simulink model "W06_3_heading"  (R2024b)
settings: Solver=FixedStepDiscrete  StartTime=0.0  StopTime=inf  FixedStep=0.05  RelTol=1e-3
libraries: ros2lib x5, slpidlib x1
settings Model: Creator=admin  LastModifiedBy=admin

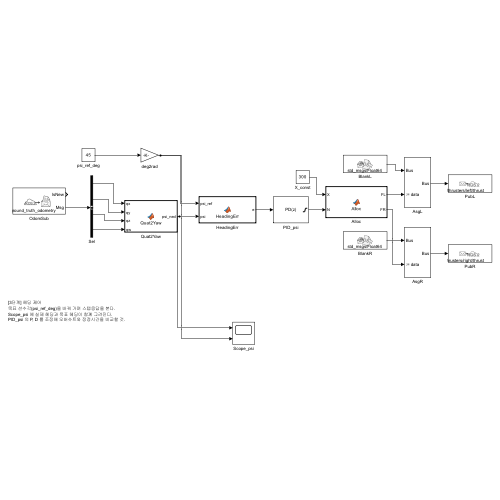
[thumbnail: Simulink's stored preview of the top-level diagram]
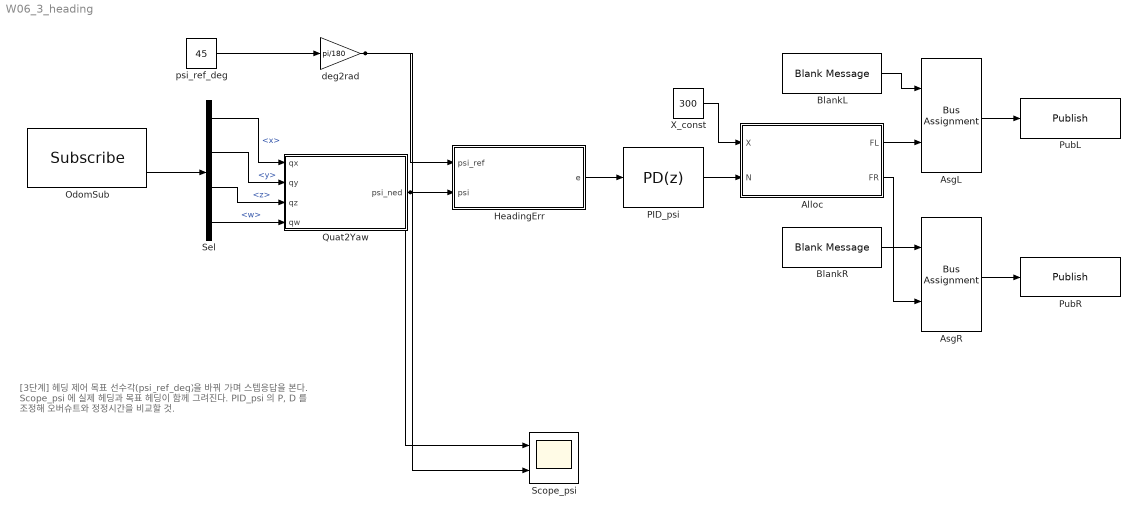
== system W06_3_heading ==
  note: [3단계] 헤딩 제어
      | 목표 선수각(psi_ref_deg)을 바꿔 가며 스텝응답을 본다.
      | Scope_psi 에 실제 헤딩과 목표 헤딩이 함께 그려진다.
      | PID_psi 의 P, D 를 조정해 오버슈트와 정정시간을 비교할 것.
  Alloc : MATLAB Function  TreatAsAtomicUnit=on
  AsgL : BusAssignment  AssignedSignals=data
  AsgR : BusAssignment  AssignedSignals=data
  BlankL : ros2lib/Blank Message  messageClass=Message  entityType=std_msgs/Float64  messageType=std_msgs/Float64  SampleTime=0.05
  BlankR : ros2lib/Blank Message  messageClass=Message  entityType=std_msgs/Float64  messageType=std_msgs/Float64  SampleTime=0.05
  HeadingErr : MATLAB Function  TreatAsAtomicUnit=on
  OdomSub : ros2lib/Subscribe  topicSource=Specify your own  topic=/wamv/sensors/position/ground_truth_odometry  messageType=nav_msgs/Odometry  sampleTime=0.05  QOSHistory=Keep last  QOSDepth=1  QOSReliability=Reliable  QOSDurability=Volatile  QOSDeadline=Inf  QOSLifespan=Inf  QOSLiveliness=Automatic  QOSLeaseDuration=Inf  QOSAvoidROSNamespaceConventions=off
  PID_psi : slpidlib/PID Controller  Controller=PD  Form=Parallel  TimeDomain=Discrete-time  UseExternalTs=off  SampleTime=0.05  IntegratorMethod=Forward Euler  FilterMethod=Forward Euler  ControllerParametersSource=internal  P=800  I=1  UseKiTs=off  D=400  UseExternalDerivativeSource=off  N=100  UseFilter=on  TunerSelectOption=Transfer Function Based (PID Tuner App)  InitialConditionSource=internal  InitialConditionForIntegrator=0  InitialConditionForFilter=0  DifferentiatorICPrevScaledInput=0  ExternalReset=none  TrackingMode=off  Kt=1  LimitOutput=on  SatLimitsSource=internal  UpperSaturationLimit=500  LowerSaturationLimit=-500  LinearizeAsGain=off  AntiWindupMode=none  Kb=1  LimitIntegrator=off  UpperIntegratorSaturationLimit=inf  LowerIntegratorSaturationLimit=-inf  POutMin=[]  POutMax=[]  IOutMin=[]  IOutMax=[]  DOutMin=[]  DOutMax=[]  NOutMin=[]  NOutMax=[]  SumOutMin=[]  SumOutMax=[]  SaturationOutMin=[]  SaturationOutMax=[]  PParamMin=[]  PParamMax=[]  IParamMin=[]  IParamMax=[]  DParamMin=[]  DParamMax=[]  NParamMin=[]  NParamMax=[]  KbParamMin=[]  KbParamMax=[]  KtParamMin=[]  KtParamMax=[]  KbOutMin=[]  KbOutMax=[]  KtOutMin=[]  KtOutMax=[]  IntegratorOutMin=[]  IntegratorOutMax=[]  FilterOutMin=[]  FilterOutMax=[]  SumI1OutMin=[]  SumI1OutMax=[]  SumI2OutMin=[]  SumI2OutMax=[]  SumI3OutMin=[]  SumI3OutMax=[]  SumI4OutMin=[]  SumI4OutMax=[]  SumDOutMin=[]  SumDOutMax=[]  DifferentiatorOutMin=[]  DifferentiatorOutMax=[]  FilterDiffOutCoefMin=[]  FilterDiffOutCoefMax=[]  ReciprocalOutMin=[]  ReciprocalOutMax=[]  SumDenOutMin=[]  SumDenOutMax=[]  SumNumOutMin=[]  SumNumOutMax=[]  DivideOutMin=[]  DivideOutMax=[]  UdiffTsProdOutMin=[]  UdiffTsProdOutMax=[]  NTsProdOutMin=[]  NTsProdOutMax=[]  UintegralTsProdOutMin=[]  UintegralTsProdOutMax=[]  UngainTsProdOutMin=[]  UngainTsProdOutMax=[]  ClampingZeroOutDataTypeStr=Inherit: Inherit via back propagation  ClampingZeroOutMin=[]  ClampingZeroOutMax=[]  FilterDenConstantOutDataTypeStr=Inherit: Inherit via back propagation  FilterDenConstantOutMin=[]  FilterDenConstantOutMax=[]  PCopyOutDataTypeStr=Inherit: Inherit via back propagation  PCopyOutMin=[]  PCopyOutMax=[]  NCopyOutDataTypeStr=Inherit: Inherit via back propagation  NCopyOutMin=[]  NCopyOutMax=[]  IntegratorContinuousStateAttributes=''  IntegratorStateMustResolveToSignalObject=off  IntegratorRTWStateStorageClass=Auto  FilterContinuousStateAttributes=''  FilterStateMustResolveToSignalObject=off  FilterRTWStateStorageClass=Auto  ParallelPVariant=InternalParameters  IdealPVariant=Disabled  IVariant=Disabled  DVariant=InternalParameters  IntegratorVariant=Disabled  SatVariant=Enabled  AWVariant=Disabled  PCopyVariant=Disabled  TRVariant=Disabled  FdbkBlocksVariant=Forward  IdealPFdbkVariant=Disabled  SatFdbkVariant=Disabled  DerivativeFilterVariant=ForwardEulerFilter  NVariant=InternalParameters  NCopyVariant=Disabled  FilterICVariant=InternalICsFilter  IntegratorICVariant=Disabled  ExternalResetVariant=Disabled  TRSumVariant=Passthrough  SumFdbkVariant=Disabled  SumVariant=Sum_PD  TsampFilterVariant=InternalTs  TsampNgainVariant=Passthrough  TsampIntegralVariant=Disabled_SignalSpec  ExternalSaturationOutDataTypeStr=Inherit: Same as second input  DerivativeSourceVariant=ErrorSignal  PreIntVariant=InternalPreInt
      settings: LibrarySourceBlock=simulink/Discrete/Discrete PID Controller
  PubL : ros2lib/Publish  topicSource=Specify your own  topic=/wamv/thrusters/left/thrust  messageType=std_msgs/Float64  QOSHistory=Keep last  QOSDepth=1  QOSReliability=Reliable  QOSDurability=Volatile  QOSDeadline=Inf  QOSLifespan=Inf  QOSLiveliness=Automatic  QOSLeaseDuration=Inf  QOSAvoidROSNamespaceConventions=off
  PubR : ros2lib/Publish  topicSource=Specify your own  topic=/wamv/thrusters/right/thrust  messageType=std_msgs/Float64  QOSHistory=Keep last  QOSDepth=1  QOSReliability=Reliable  QOSDurability=Volatile  QOSDeadline=Inf  QOSLifespan=Inf  QOSLiveliness=Automatic  QOSLeaseDuration=Inf  QOSAvoidROSNamespaceConventions=off
  Quat2Yaw : MATLAB Function  TreatAsAtomicUnit=on
  Scope_psi : Scope  NumInputPorts=2
  Sel : BusSelector  OutputSignals=pose.pose.orientation.x,pose.pose.orientation.y,pose.pose.orientation.z,pose.pose.orientation.w
  X_const : Constant  Value=300
  deg2rad : Gain  Gain=pi/180
  psi_ref_deg : Constant  Value=45
  wires:
  OdomSub/2 -> Sel/1
  psi_ref_deg/1 -> deg2rad/1
  Alloc/2(FR) -> AsgR/2
  deg2rad/1 -> HeadingErr/1(psi_ref), Scope_psi/2
  Sel/1 -> Quat2Yaw/1(qx)  "<x>"
  AsgL/1 -> PubL/1
  X_const/1 -> Alloc/1(X)
  Sel/2 -> Quat2Yaw/2(qy)  "<y>"
  Sel/3 -> Quat2Yaw/3(qz)  "<z>"
  Sel/4 -> Quat2Yaw/4(qw)  "<w>"
  Quat2Yaw/1(psi_ned) -> HeadingErr/2(psi), Scope_psi/1
  HeadingErr/1(e) -> PID_psi/1
  PID_psi/1 -> Alloc/2(N)
  BlankL/1 -> AsgL/1
  Alloc/1(FL) -> AsgL/2
  BlankR/1 -> AsgR/1
  AsgR/1 -> PubR/1

== matlab function W06_3_heading/HeadingErr ==
  data: psi_ref input; e output; psi input
function e = HeadingErr(psi_ref, psi)
%#codegen
% Shortest angular difference, wrapped to [-pi, pi]
d = psi_ref - psi;
e = atan2(sin(d), cos(d));

== matlab function W06_3_heading/Quat2Yaw ==
  data: qx input; psi_ned output; qy input; qz input; qw input
function psi_ned = Quat2Yaw(qx, qy, qz, qw)
%#codegen
% ROS quaternion (ENU body) -> NED heading [rad]
yaw_enu = atan2(2*(qw*qz + qx*qy), 1 - 2*(qy*qy + qz*qz));
psi = pi/2 - yaw_enu;
psi_ned = atan2(sin(psi), cos(psi));   % wrap to [-pi, pi]

== matlab function W06_3_heading/Alloc ==
  data: X input; FL output; N input; FR output
function [FL, FR] = Alloc(X, N)
%#codegen
% Differential thrust allocation for the 2-thruster WAM-V
%   X : surge force  [N]
%   N : yaw moment   [N*m], positive turns to starboard
B_half = 1.027135;      % half distance between thrusters [m]
Fmax   = 250;           % thrust limit per thruster [N]
FL = X/2 + N/(2*B_half);
FR = X/2 - N/(2*B_half);
FL = max(min(FL, Fmax), -Fmax);
FR = max(min(FR, Fmax), -Fmax);
